simulink model "motorSimulator"  (R2021a)
settings: Solver=VariableStepAuto  StartTime=0.0  StopTime=10.0  RelTol=1e-3
settings Model: Creator=iumrikhin  LastModifiedBy=iumrikhin

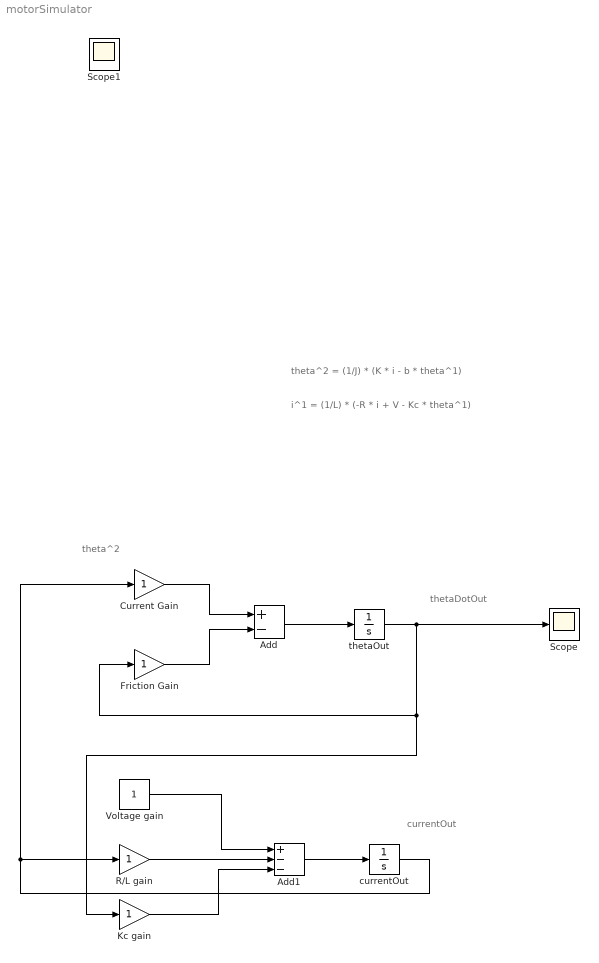
== system motorSimulator ==
  note: currentOut
  note: thetaDotOut
  note: theta^2
  note: i^1 = (1/L) * (-R * i + V - Kc * theta^1)
  note: theta^2 = (1/J) * (K * i - b * theta^1)
  Add : Sum  Inputs=+-
  Add1 : Sum  Inputs=+--
  Current Gain : Gain
  Friction Gain : Gain
  Kc gain : Gain
  R/L gain : Gain
  Scope : Scope
  Voltage gain : Constant
  currentOut : Integrator
  thetaOut : Integrator
  Scope1 : Scope
  wires:
  thetaOut/1 -> Scope/1, Kc gain/1, Friction Gain/1
  Current Gain/1 -> Add/1
  Friction Gain/1 -> Add/2
  Add/1 -> thetaOut/1
  Voltage gain/1 -> Add1/1
  R/L gain/1 -> Add1/2
  Kc gain/1 -> Add1/3
  Add1/1 -> currentOut/1
  currentOut/1 -> R/L gain/1, Current Gain/1
